simulink model "SamsonAntrieb_MdlIdent"  (R2017a)
settings: Solver=VariableStepAuto  StartTime=0.0  StopTime=67  FixedStep=0.001  MaxStep=1e-2  RelTol=1e-6  EnableMultiTasking=on
undefined symbols (not defined in the file or in its folder): mdlPara
libraries: PASL_Models x1, PASL_Tools x1
settings Model: Creator=fbwk  LastModifiedBy=mmnt
settings SolverCC: SolverResetMethod=Robust
settings DataIOCC: LimitDataPoints=on  SaveFormat=Array  SaveOutput=off  SignalLogging=off  DSMLogging=off  SaveTime=off
settings OptimizationCC: LifeSpan=inf
settings DebuggingCC: SolverPrmCheckMsg=warning  SFUnexpectedBacktrackingDiag=warning  SFNoUnconditionalDefaultTransitionDiag=warning  SFExecutionAtInitializationDiag=none
settings HardwareCC: ProdBitPerPointer=32  ProdBitPerSizeT=32  ProdBitPerPtrDiffT=32  ProdLargestAtomicFloat=None  ProdIntDivRoundTo=Undefined  ProdEndianess=Unspecified  ProdWordSize=32  ProdHWDeviceType=32-bit Generic
settings ModelReferenceCC: PropagateSignalLabelsOutOfModel=off
settings GRTTargetCC: TargetLangStandard=C89/C90 (ANSI)  GeneratePreprocessorConditionals=Disable all
settings ConfigComp: CovMetricSettings=dw  CovHtmlReporting=on  CovSaveCumulativeToWorkspaceVar=on  CovSaveSingleToWorkspaceVar=on  CovExternalEMLEnable=off  CovSFcnEnable=off

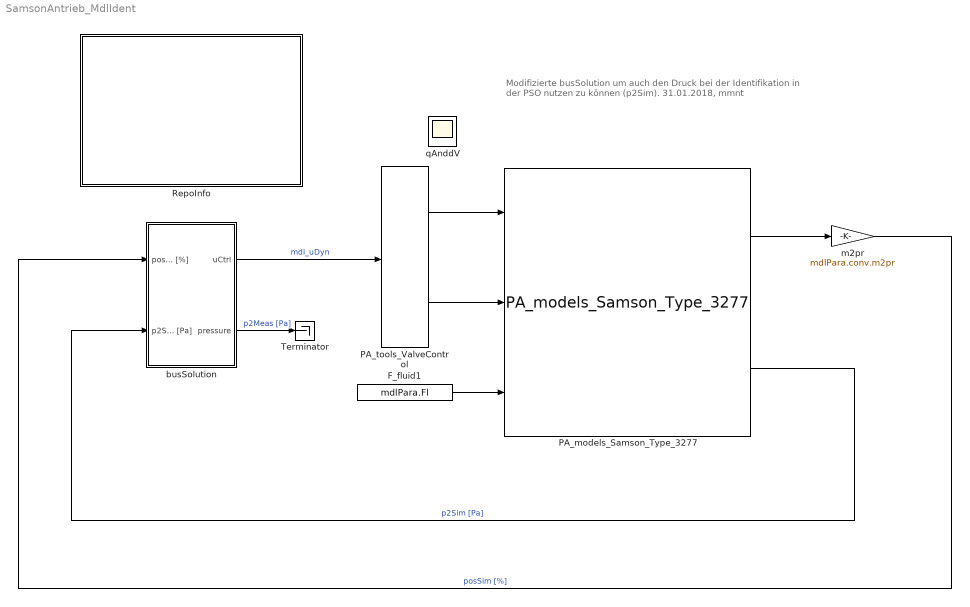
== system SamsonAntrieb_MdlIdent ==
  note: Modifizierte busSolution um auch den Druck bei der Identifikation
      | in der PSO nutzen zu können (p2Sim).
      | 31.01.2018, mmnt
  F_fluid1 : Constant  Value=mdlPara.Fl
  PA_models_Samson_Type_3277 : PASL_Models/PA_models_Samson_Type_3277  Tag=PA_models_CMSI_piston_singleActing  mdlPara=mdlPara
      settings: SourceProductName=PASL
  PA_tools_ValveControl : PASL_Tools/PA_tools_ValveControl
      settings: SourceProductName=PASL
  RepoInfo : Subsystem  Tag=RevTagSubSys  AncestorBlock=PASL_Tools/RepoInfo  mask(cover){}
      mask help: mask for library reasons
      settings: OpenFcn=PA_setRepoInfoBlock()
      mask Display: text(.05,.95,'Project:\n   Rev#:  34\n   RevID: edff4ab12a1e\n   date:  Mon Jan 29 17:36:46 2018 +0100\n\nPASL:\n   Rev#:  456\n   RevID: 2bc290b3a386\n   date:  Mon Jan 29 08:53:47 2018 +0100\n\nPATL:\n   Rev#:  75\n   RevID: e9f2d7fd98d6\n   date:  Mon Jan 29 09:04:49 2018 +0100','hor','left','ver','top')
  Terminator : Terminator
  busSolution : Subsystem  VariantControl=busVariant
  m2pr : Gain  Gain=mdlPara.conv.m2pr  OutDataTypeStr=single
  qAnddV : Scope
  wires:
  m2pr/1 -> busSolution/1(posSim [%])  "posSim [%]"
  busSolution/1(uCtrl) -> PA_tools_ValveControl/1  "mdl_uDyn"
  PA_models_Samson_Type_3277/2 -> busSolution/2(p2Sim [Pa])  "p2Sim [Pa]"
  PA_tools_ValveControl/1 -> PA_models_Samson_Type_3277/1
  PA_tools_ValveControl/2 -> PA_models_Samson_Type_3277/2
  busSolution/2(pressure) -> Terminator/1  "p2Meas [Pa]"
  PA_models_Samson_Type_3277/1 -> m2pr/1
  F_fluid1/1 -> PA_models_Samson_Type_3277/3

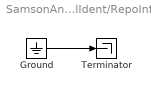
== system SamsonAntrieb_MdlIdent/RepoInfo ==
  Ground : Ground
  Terminator : Terminator
  wires:
  Ground/1 -> Terminator/1

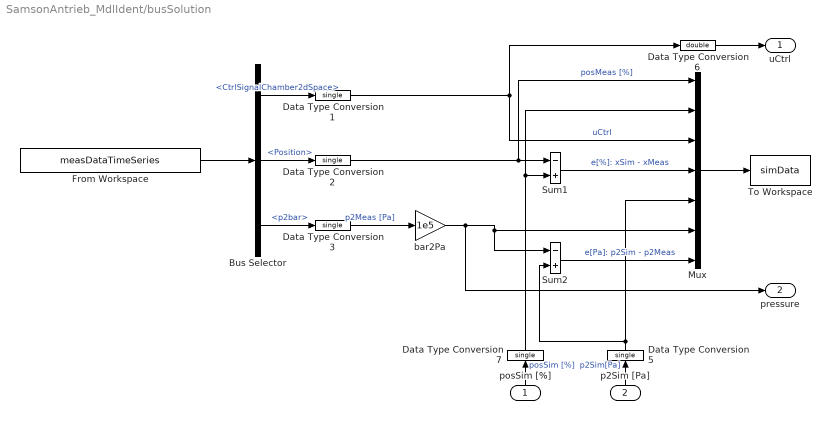
== system SamsonAntrieb_MdlIdent/busSolution ==
  posSim [%] : Inport
  p2Sim [Pa] : Inport  Port=2
  Bus Selector : BusSelector  OutputSignals=CtrlSignalChamber2dSpace,Position,p2bar
  Data Type Conversion{1..3,5,7} (5 alike) : DataTypeConversion  OutDataTypeStr=single
  Data Type Conversion6 : DataTypeConversion  OutDataTypeStr=double
  From Workspace : FromWorkspace  VariableName=measDataTimeSeries  OutDataTypeStr=Bus: busMeasData  SampleTime=0
  Mux : Mux  Inputs=7
  Sum1 : Sum  Inputs=-+
  Sum2 : Sum  Inputs=-+
  To Workspace : ToWorkspace  VariableName=simData  SaveFormat=Structure With Time  SampleTime=-1
  bar2Pa : Gain  Gain=1e5
  uCtrl : Outport
  pressure : Outport  Port=2
  wires:
  Bus Selector/3 -> Data Type Conversion3/1  "<p2bar>"
  Bus Selector/1 -> Data Type Conversion1/1  "<CtrlSignalChamber2dSpace>"
  From Workspace/1 -> Bus Selector/1
  Bus Selector/2 -> Data Type Conversion2/1  "<Position>"
  posSim [%]/1 -> Data Type Conversion7/1  "posSim [%]"
  Sum1/1 -> Mux/4  "e[%]: xSim - xMeas"
  Mux/1 -> To Workspace/1
  Data Type Conversion1/1 -> Mux/3, Data Type Conversion6/1  "uCtrl"
  Data Type Conversion2/1 -> Sum1/1, Mux/1  "posMeas [%]"
  Data Type Conversion3/1 -> bar2Pa/1  "p2Meas [Pa]"
  p2Sim [Pa]/1 -> Data Type Conversion5/1  "p2Sim[Pa]"
  Sum2/1 -> Mux/7  "e[Pa]: p2Sim - p2Meas"
  Data Type Conversion6/1 -> uCtrl/1
  Data Type Conversion7/1 -> Mux/2, Sum1/2
  Data Type Conversion5/1 -> Mux/5, Sum2/2
  bar2Pa/1 -> pressure/1, Sum2/1, Mux/6
